simulink model "M_FLCC"  (R2022a)
settings: Solver=ode4  StartTime=0.0  StopTime=100  FixedStep=0.01  RelTol=1e-3
PreLoadFcn:
  | load('BUS_STRUCTURE_FLCC.mat');
InitFcn:
  | load('BUS_STRUCTURE_FLCC.mat');
undefined symbols (not defined in the file or in its folder): f16data
libraries: sharedtransform x6, simulink_extras x4, aerolibatmos2 x1
(part 2 of 2)

== matlab function M_FLCC/FlightController/AttitudeOuterLoop/Auto_Longitudinal/PITCH_AGCAS_PARS/HoldHeight/fcnQuatAttitudeController ==
  data: quat input; qCmd output; quat_sp input; pqr input; beta input; tick input; dt input
function qCmd = fcnQuatAttitudeController(quat, quat_sp, pqr, beta, tick, dt)
%fcnQuatAttitudeController
%
% -- Input --
% quat : quaternion vector (1-by-4 column vector of real numbers)
% quat_sp : (set point) quaternion vector (1-by-4 column vector of real numbers)
% -- Output --
% pqrCmd : angular rate command (3-by-1 column vector of real numbers)

persistent firstRun prev_quat_err prevTick
if isempty(prev_quat_err)
    prev_quat_err = [1, 0, 0, 0];
end
if isempty(firstRun)
    firstRun = true;
end
if isempty(prevTick)
    prevTick = uint32(0);
end

% Initialize Integral control term
if (tick - prevTick ) >= uint32(2)
    prev_quat_err = [1, 0, 0, 0];
end

% Intialize
qCmd = 0.0;
quat_err = zeros(1,4);
eul_ypr = zeros(1,3);

% Controller gain
Kp_p = 2.0;
Kp_q = 0.2;
Kd_q = -0.01;
% Kd_q = -0.0;
Kp_r = 0.0;
Kp_beta = -0.03;
D2R = pi/180;

% Attitude error quaternion
quat_err = quatmultiply( quatconj(quat'), quat_sp' );
quat_err = quatnormalize(quat_err);

% Convert a quat_err to axis-angle representation
ang_err = 2 * acos(quat_err(1));
if ( (IsNear(quat_err(1), 1)) || (IsNear(quat_err(1), -1)) )
    u_x = 0.0;
    u_y = 0.0;
    u_z = 0.0;
else
    u_x = quat_err(2) / sqrt(1 - quat_err(1)^2);
    u_y = quat_err(3) / sqrt(1 - quat_err(1)^2);
    u_z = quat_err(4) / sqrt(1 - quat_err(1)^2);
end

% % Choose a shorter rotation ang_err
if (ang_err > pi)
    ang_err = abs(ang_err - 2*pi);
    u_x = -u_x;
    u_y = -u_y;
    u_z = -u_z;
else
end

% Convert the new attitude error from the axis-angle representation back
% to quaternion form
quat_err(1) = cos(ang_err/2);
quat_err(2) = u_x * sin(ang_err/2);
quat_err(3) = u_y * sin(ang_err/2);
quat_err(4) = u_z * sin(ang_err/2);

eul_ypr = quat2eul(quat', 'ZYX');
% % Ensure we have shorter rotation
if (quat_err(1) < 0)
    quat_err(1) = -quat_err(1);
    quat_err(2) = -quat_err(2);
    quat_err(3) = -quat_err(3);
    quat_err(4) = -quat_err(4);
else
end

% Normalize 
quat_err = quatnormalize(quat_err);

% Euler angles from quaternion
eul_ypr = quat2eul(quat', 'ZYX');
rol = eul_ypr(3);
pit = eul_ypr(2);

% Inversion from attitude kinematics
q = pqr(2);
r = pqr(3);

if abs(pit) > 80*D2R
    pTrim = 0;
    qTrim = 0;
else
    pTrim  =  (- (q * sin(rol) * tan(pit)) - (r * cos(rol) * tan(pit)));
    qTrim  =  (   r * tan(rol));
end
% rTrim  =  (   qTrim / tan(phi));
rTrim  = 0;

% Calculate angular rate command
if (firstRun)
    DTerm = [1, 0, 0, 0];
else
    DTerm = (quat_err - prev_quat_err)/dt;
    DTerm(3) = fcnSaturation(DTerm(3), 0.1);
end
pCmd = pTrim + 2 * Kp_p * quat_err(2);
qCmd = qTrim + 2 * Kp_q * quat_err(3) + Kd_q * DTerm(3);
rCmd = rTrim + 2 * Kp_r * quat_err(4) + Kp_beta * (0 - beta);
% pCmd = K_p * quat_err(2);
% qCmd = K_q * quat_err(3);
% rCmd = rTrim + 2 * K_r * quat_err(4) + Kbeta * (0 - beta);


% Saturate command
plim = 25 * D2R;
qlim = 25 * D2R;
rlim = 20 * D2R;

pCmd = fcnSaturation(pCmd, plim);
qCmd = fcnSaturation(qCmd, qlim);
rCmd = fcnSaturation(rCmd, rlim);

% Output
pqrCmd = [pCmd; qCmd; rCmd];

firstRun = false;
prev_quat_err = quat_err;
prevTick = tick;
end


function in = fcnSaturation(in, lim)

if abs(in)>lim
    in = lim*sign(in);
end

end

== matlab function M_FLCC/FlightController/LeadingEdgeFlapScheduler ==
  data: groundStage input; lefDeg output; alpha input; Ps input; qBar input; lefDegRaw output
function [lefDeg, lefDegRaw]= LeadingEdgeFlapScheduler(groundStage, alpha, Ps, qBar)
%LeadingEdgeFlapScheduler 앞전플랩 명령을 계산한다
% --- INPUT ---
% groundStage: 지상 운동 단계
% ALPHA: 받음각 (deg)
% Ps: 정압 (Pa)
% qBar: 동압 (Pa)
% --- OUTPUT ---
% lefDeg: 앞전플랩 명령 (deg)

% Initialize output
lefDeg = 0.0;
RAD2DEG = 180/pi;

if ( (groundStage >= uint8(2)) && (groundStage <= uint8(5)) )
    % 50%
    lefDeg = 12.5;
else
    if abs(qBar) < 0.1
        lefDeg = 0.0;
    else
        lefDeg = 1.38 * (alpha*RAD2DEG) - 9.05 * (Ps/qBar) + 1.45;
    end
end
lefDegRaw = lefDeg;
lefDeg = fcnSaturation(lefDeg, 0, 25);

end

function out = fcnSaturation(in, lower, upper)

if in > upper
    out = upper;
elseif in < lower
    out = lower;
else
    out = in;
end

end

== matlab function M_FLCC/FlightController/ThrustController/FLCC_CalculateDrag ==
  data: CX input; D output; qBar input; Sref input
function D = CalculateDrag(CX, qBar, Sref)

D = -CX*qBar*Sref;

end

== matlab function M_FLCC/FlightController/ThrustController/FLCC_VelController ==
  data: VtCmd input; Throttle_Cmd output; DYN_STATE input; D input; m input; dt input
function Throttle_Cmd = VelController(VtCmd, DYN_STATE, D, m, dt)
persistent intVtc_Vt prevVtc_Vt
if isempty(intVtc_Vt)
    intVtc_Vt  = 0.0;
    prevVtc_Vt = 0.0;
end

% Constants & Macros
GRAV = 9.8;
DEG2RAD = pi/180;

Vt = DYN_STATE.Vt;
the = DYN_STATE.pitch;
alp = DYN_STATE.alpha;
gam = the - alp;

Vtc_Vt = VtCmd - Vt;
intVtc_Vt  = ( intVtc_Vt + (prevVtc_Vt + Vtc_Vt)*dt/2 );
LimIntVtc_Vt = 50;
intVtc_Vt = fcnSaturation(intVtc_Vt, -LimIntVtc_Vt, LimIntVtc_Vt);
prevVtc_Vt = Vtc_Vt;

% FtTrim = 1/cos(alp)*(D + m*Grav*sin(gam));
% FtTerm1 = wn_Vt^2*m/cos(alp)*intVtc_Vt;
% FtTerm2 = -2*Zeta_Vt*wn_Vt*m/cos(alp)*Vt;

tauVt = 0.28;
intVt = 1.2;

if ( abs(alp) < 85*DEG2RAD )
    Kp  = m/tauVt/cos(alp);
else
    Kp  = m/tauVt/cosd(85);
end
Ki  = intVt;
FtTrimD = 1/cos(alp)*(D); 
FtTrimM = 1/cos(alp)*(m*GRAV*sin(gam));
FtTerm1 = Kp*Vtc_Vt;
FtTerm2 = Ki*intVtc_Vt;

FtCmd   = FtTrimD + FtTrimM + FtTerm1 + FtTerm2;

Ft_lb = fcnSaturation(FtCmd / 4.448, 1000, 29000);
Throttle_Cmd = thrust2thtl(Ft_lb);


end


function out = fcnSaturation(in, lower, upper)

if in > upper
    out = upper;
elseif in < lower
    out = lower;
else
    out = in;
end

end

function thtl = thrust2thtl(thrust_lb)
pow = thrust_lb / 29000;

if (pow <= 0.50)
    thtl = pow / 0.6494;
else
    thtl = (1.1738 + pow) / 2.1738;
end
end

== matlab function M_FLCC/FlightController/AttitudeOuterLoop/Auto_LateralDirectional/fcnQuatAttitudeController ==
  data: quat input; pCmd output; quat_sp input; pqr input; beta input; tick input; dt input; rCmd output
function [pCmd, rCmd] = fcnQuatAttitudeController(quat, quat_sp, pqr, beta, tick, dt)
%fcnQuatAttitudeController
%
% -- Input --
% quat : quaternion vector (1-by-4 column vector of real numbers)
% quat_sp : (set point) quaternion vector (1-by-4 column vector of real numbers)
% -- Output --
% pqrCmd : angular rate command (3-by-1 column vector of real numbers)

persistent firstRun prev_quat_err prevTick
if isempty(prev_quat_err)
    prev_quat_err = [1, 0, 0, 0];
end
if isempty(firstRun)
    firstRun = true;
end
if isempty(prevTick)
    prevTick = uint32(0);
end

% Initialize Integral control term
if (tick - prevTick ) >= uint32(2)
    prev_quat_err = [1, 0, 0, 0];
end

% Intialize
pCmd = 0.0;
rCmd = 0.0;
quat_err = [1, 0, 0, 0];
eul_ypr = zeros(1,3);

% Controller gain
Kp_p = 2.0;
Kp_r = 0.0;
Kp_beta = -0.5;
D2R = pi/180;

% Attitude error quaternion
quat_err = quatmultiply( quatconj(quat'), quat_sp' );
quat_err = quatnormalize(quat_err);

% Convert a quat_err to axis-angle representation
ang_err = 2 * acos(quat_err(1));
if ( (IsNear(quat_err(1), 1)) || (IsNear(quat_err(1), -1)) )
    u_x = 0.0;
    u_y = 0.0;
    u_z = 0.0;
else
    u_x = quat_err(2) / sqrt(1 - quat_err(1)^2);
    u_y = quat_err(3) / sqrt(1 - quat_err(1)^2);
    u_z = quat_err(4) / sqrt(1 - quat_err(1)^2);
end

% % Choose a shorter rotation ang_err
if (ang_err > pi)
    ang_err = abs(ang_err - 2*pi);
    u_x = -u_x;
    u_y = -u_y;
    u_z = -u_z;
else
end

% Convert the new attitude error from the axis-angle representation back
% to quaternion form
quat_err(1) = cos(ang_err/2);
quat_err(2) = u_x * sin(ang_err/2);
quat_err(3) = u_y * sin(ang_err/2);
quat_err(4) = u_z * sin(ang_err/2);

eul_ypr = quat2eul(quat', 'ZYX');
% % Ensure we have shorter rotation
if (quat_err(1) < 0)
    quat_err(1) = -quat_err(1);
    quat_err(2) = -quat_err(2);
    quat_err(3) = -quat_err(3);
    quat_err(4) = -quat_err(4);
else
end

% Normalize 
quat_err = quatnormalize(quat_err);

% Euler angles from quaternion
eul_ypr = quat2eul(quat', 'ZYX');
rol = eul_ypr(3);
pit = eul_ypr(2);

% Inversion from attitude kinematics
p = pqr(1);
q = pqr(2);
r = pqr(3);

if abs(pit) > 80*D2R
    pTrim = 0;
else
    pTrim  =  (- (q * sin(rol) * tan(pit)) - (r * cos(rol) * tan(pit)));
end
rTrim  = 0;

pCmd = pTrim + 2 * Kp_p * quat_err(2);
rCmd = rTrim + 2 * Kp_r * quat_err(4) + Kp_beta * (0 - beta);

% Saturate command
plim = 25 * D2R;
rlim = 20 * D2R;
pCmd = fcnSaturation(pCmd, plim);
rCmd = fcnSaturation(rCmd, rlim);

firstRun = false;
prev_quat_err = quat_err;
prevTick = tick;

end


function in = fcnSaturation(in, lim)

if abs(in)>lim
    in = lim*sign(in);
end

end

== matlab function M_FLCC/FlightController/AttitudeOuterLoop/Manual_Longitudinal/Manual_Long ==
  data: STICK input; qCmd output; DYN_STATE input
function qCmd = Manual_Long(STICK, DYN_STATE)
%Manual_Long
% --- Input ---
% --- Output ---
% qCmd: angular rate command along body y-axis

% Intialize output
qCmd = 0.0;

% Rearrange input
rol = DYN_STATE.roll;
pit = DYN_STATE.pitch;
q = DYN_STATE.omY;
r = DYN_STATE.omZ;
pitchStick = STICK.pitchStick;
expo = 0.5;

if ( -0.05 <= pitchStick ) && ( pitchStick <= 0.05 )
    pitchStick = 0;
else
    pitchStick = (expo*pitchStick^3 + (1-expo)*pitchStick);
end


% Stick
pitchStick = fcnSaturation(pitchStick, 1);

% Controller gain
Kp_q_stick = 0.3;
D2R = pi/180;

if abs(pit) > 80*D2R
    qTrim = 0.0;
else
    qTrim  =  (   r * tan(rol));
end

% Calculate angular rate command
qCmd = qTrim + Kp_q_stick * pitchStick;

% Saturate command
qlim = 25 * D2R;
qCmd = fcnSaturation(qCmd, qlim);

end


function in = fcnSaturation(in, lim)

if abs(in)>lim
    in = lim*sign(in);
end

end

== matlab function M_FLCC/FlightController/AttitudeOuterLoop/Auto_Longitudinal/PITCH_AGCAS_PARS/RecoveryPullUp/GetQCmdATF ==
  data: azCmd input; az input; qCmd output; Vt input; tick input; dt input
function qCmd   = GetQCmdATF(azCmd, az, Vt, tick, dt)
%GetQCmdATF
% == INPUT
% azCmd     : Acceleration Z Command (m/s^2)
% az        : Acceleration Z (m/s^2)
% q         : pitch rate (rad/s)
% U0        : Velocity X (m/s)
% dt        : time interval (sec)
% == OUTPUT
% qCmd      : pitch rate command (rad/s)

persistent zeta wn d2r azInt qInt

if isempty(zeta)
    zeta = 0.70;
end
if isempty(wn)
    wn = 6.3;
end
if isempty(d2r)
    d2r = pi/180;
end
if isempty(azInt)
    azInt = 0.0;
end
if isempty(qInt)
    qInt = 0.0;
end

% Initialize 
qCmd = 0.0;

% Pitch angular velocity command shaping ( azCmd -> qCmd )
Kp_az = - 1 / Vt;
Ki_az = - 1 * 0.05 / Vt;

azInt = azInt + (azCmd - az) * dt;
azInt = fcnSaturation(azInt, 20.0);

qCmd = Kp_az * azCmd + Kp_az * (azCmd - az) + Ki_az * azInt;
end

function out = fcnSaturation(in, lim)

if abs(in) > lim
    out = sign(in)*lim;
else
    out = in;
end

end

== matlab function M_FLCC/FlightController/AttitudeOuterLoop/Auto_Longitudinal/PITCH_AGCAS_PARS/ConfigRecoveryStage ==
  data: prevStage input; curStage output; rollRad input; FPARad input; maxFPARad input
function curStage = ConfigRecoveryStage(prevStage, rollRad, FPARad, maxFPARad)
%ConfigRecoveryStage
% Recovery Stage
% 0: At start / or the end
% 1: Roll Recovering
% 2: Roll Recovered. 5G Pull-Up
% 3: Max Flight Path Angle Reached
% 4: Level Recovering
% 5: Level Recovered

persistent timeSpentMaxFPA dt timeSpentLevelRecovering

if (isempty(dt))
    dt = 0.04;
end
if (isempty(timeSpentMaxFPA))
    timeSpentMaxFPA = 0.0;
end
if (isempty(timeSpentLevelRecovering))
    timeSpentLevelRecovering = 0.0;
end

% Constant
DEG2RAD = pi/180;

curStage = prevStage;

if (prevStage == uint8(0))
    curStage = uint8(1);
    timeSpentMaxFPA = 0.0;
    timeSpentLevelRecovering = 0.0;
else
end

maxFPARad = saturate(maxFPARad, 45*DEG2RAD, 85*DEG2RAD);

if ( (prevStage == uint8(1)) || (curStage == uint8(1)) )
    % Roll 안정화가 되면 2로
    if (rollRad < 0.5*DEG2RAD)
        curStage = uint8(2);
    end

elseif (prevStage == uint8(2))
    % Max Flight Path Angle 도달하면, 3으로
    if ( FPARad > maxFPARad )
        curStage = uint8(3);
    end

elseif (prevStage == uint8(3))
    % 최대 비행경로각 도달 후 10초가 경과하면, 4로
    if (timeSpentMaxFPA > 10.0)
        curStage = uint8(4);
        timeSpentMaxFPA = 0.0;
    else
        timeSpentMaxFPA = timeSpentMaxFPA + dt;
    end

elseif (prevStage == uint8(4))
    
    if (timeSpentLevelRecovering > 5.0)
        curStage = uint8(5);
    end
    timeSpentLevelRecovering = timeSpentLevelRecovering + dt;

elseif (prevStage == uint8(5))

    curStage = uint8(0);

end

end


function outVal = saturate(inVal, minVal, maxVal)

outVal = max(minVal, min(inVal, maxVal));

end

== matlab function M_FLCC/FlightController/AttitudeOuterLoop/Auto_Longitudinal/PITCH_AGCAS_PARS/ConfigStageChange ==
  data: curStage input; prevStage input; isStageChanged output
function isStageChanged  = ConfigStageChange(curStage, prevStage)
%ConfigureStageChange

isStageChanged = false;

if prevStage ~= curStage
    
    isStageChanged = true;
    
else
    
end

end

== matlab function M_FLCC/FlightController/AttitudeOuterLoop/Auto_Longitudinal/PITCH_AGCAS_PARS/UpdateHeightReference ==
  data: oldhRef input; h input; newHRef output; isStageChanged input
function newHRef = UpdateHeightReference(oldhRef, h, isStageChanged)
%UpdateHeightReference

if isStageChanged == true
    
    newHRef = h;
    
else
    
    newHRef = oldhRef;
end

== matlab function M_FLCC/FlightController/AttitudeOuterLoop/Auto_Longitudinal/PITCH_ATF/GetQCmdATF ==
  data: azCmd input; az input; qCmd output; U0 input; tick input; dt input
function qCmd   = GetQCmdATF(azCmd, az, U0, tick, dt)
%GetQCmdATF
% == INPUT
% azCmd     : Acceleration Z Command (m/s^2)
% az        : Acceleration Z (m/s^2)
% q         : pitch rate (rad/s)
% U0        : Velocity X (m/s)
% dt        : time interval (sec)
% == OUTPUT
% qCmd      : pitch rate command (rad/s)

persistent zeta wn d2r azInt qInt prevTick

if isempty(zeta)
    zeta = 0.70;
end
if isempty(wn)
    wn = 6.3;
end
if isempty(d2r)
    d2r = pi/180;
end
if isempty(azInt)
    azInt = 0.0;
end
if isempty(qInt)
    qInt = 0.0;
end
if isempty(prevTick)
    prevTick = uint32(0);
end

% Initialize 
qCmd = 0.0;

if (tick - prevTick >= uint32(2))
    azInt = 0.0;
    qInt = 0.0;
end

% Vt Saturation
U0 = max(75.1089, min(U0, 500));

% Pitch angular velocity command shaping ( azCmd -> qCmd )
Kp_az = - 1.0 / U0;
Ki_az = - 1 * 0.05 / U0;

azInt = azInt + (azCmd - az) * dt;
azInt = fcnSaturation(azInt, 20.0);

qCmd = Kp_az * azCmd + Kp_az * (azCmd - az) + Ki_az * azInt;
% qCmd = Kp_az * azCmd + Kp_az * (azCmd - az) + Ki_az * azInt;
end

function out = fcnSaturation(in, lim)

if abs(in) > lim
    out = sign(in)*lim;
else
    out = in;
end

end

== matlab function M_FLCC/FlightController/AngularRateInnerLoop/fcnPQRController ==
  data: elevatorDEG output; pqrDotCmd input; ALPHA input; BETA input; pqr input; qBar input; Sref input; bref input; cref input; Cln_dar input; Clmn_trim input; inertia input; aileronDEG output; CmMat input; alpIdx input; betIdx input; deIdx1 input; dCm_dsMat input; deIdx3 input; rudderDEG output
function [elevatorDEG, aileronDEG, rudderDEG] = fcnPQRController(pqrDotCmd, ALPHA, BETA, pqr, qBar, Sref, bref, cref,...
    Cln_dar, Clmn_trim, inertia, CmMat, alpIdx, betIdx, deIdx1, dCm_dsMat, deIdx3)
% Dynamic Inversion

%% [1] Moment of inertia Matirx
Ib      = [inertia(1), -inertia(4), -inertia(5);...
          -inertia(4),  inertia(2), -inertia(6);...
          -inertia(5), -inertia(6),  inertia(3)];
%                           % Moment of inertia [kg m^2]

%% [2] Moments (L,M,N) required
% Calculate deflection command 

% Detour for divide by zero (near zero speed, dynamic pressure)
qBar = qBar + 1;
if qBar < 2
    aileronDEG = 0.0;
    rudderDEG = 0.0;
    elevatorDEG = 0.0;
    return
end

Clmn_trim = [Clmn_trim(1);Clmn_trim(2);Clmn_trim(3)];
Qinv = blkdiag( 1/(qBar * Sref * bref), 1/(qBar * Sref * cref), 1/(qBar * Sref * bref) );
M_req     = Ib*pqrDotCmd + cross(pqr, Ib*pqr);
Clmn_defl_cmd = (Qinv*M_req - Clmn_trim);

%% Calculate defelction angle of actuators
% Calculate deflection angle of aileron and rudder ( they are linear )
Cln_dar_Mat = [Cln_dar(1), Cln_dar(2);
               Cln_dar(3), Cln_dar(4)];

dadr = Cln_dar_Mat^-1*[Clmn_defl_cmd(1);Clmn_defl_cmd(3)];
aileronDEG = fcnSaturation(dadr(1), -21.5, 21.5);
rudderDEG  = fcnSaturation(dadr(2), -30, 30);
n = 1000;
% Calculate deflection angle of horizontal stabilizer (not linear, hence
% use numerical method (bisection)

elevatorDEG = bisect(Clmn_defl_cmd(2), CmMat, alpIdx, betIdx, deIdx1, dCm_dsMat, deIdx3, ALPHA, BETA, -25, 25, 0.01, n);
elevatorDEG = fcnSaturation(elevatorDEG, -25, 25);

end

function c = bisect(Cm_defl_cmd, CmMat, alpIdx, betIdx, deIdx1, dCm_dsMat, deIdx3, ALPHA, BETA, deMin, deMax, tol, n)
% Bisection method for solving the nonlinear equation  f(x)=0.
iter=0;
% fx_Upper = feval(f,a);
% fx_Lower = feval(f,b);
% fx_Upper = ( interp3(betIdx, alpIdx, deIdx1, CmMat, ALPHA, BETA, deMin) + interp2(deIdx3, alpIdx, dCm_dsMat, deMin, ALPHA) ) - Cm_defl_cmd;
% fx_Lower = ( interp3(betIdx, alpIdx, deIdx1, CmMat, ALPHA, BETA, deMax) + interp2(deIdx3, alpIdx, dCm_dsMat, deMax, ALPHA) ) - Cm_defl_cmd;
fx_Upper = ( interp3(betIdx, alpIdx, deIdx1, CmMat, BETA, ALPHA, deMin) + interp2(deIdx3, alpIdx, dCm_dsMat, deMin, ALPHA) ) - Cm_defl_cmd;
fx_Lower = ( interp3(betIdx, alpIdx, deIdx1, CmMat, BETA, ALPHA, deMax) + interp2(deIdx3, alpIdx, dCm_dsMat, deMax, ALPHA) ) - Cm_defl_cmd;
c   = (deMin + deMax)*0.5;
err = abs(deMax - deMin)*0.5;
% fprintf("fx_Upper: %f, fx_Lower: %f \r\n", fx_Upper, fx_Lower);
% disp('_____________________________________________________________________')
% disp(' iter    a            b           c           f(c)      |b-a|/2  ')
% disp('_____________________________________________________________________')
% fprintf('\n')
if (fx_Upper*fx_Lower<=0)
%     fprintf("fx_Upper: %f, fx_Lower: %f \r\n", fx_Upper, fx_Lower);

    while (err>tol)&&(iter<=n)
        % w = ( interp3(betIdx, alpIdx, deIdx1, CmMat, alp, bet, c) + interp2(deIdx3, alpIdx, dCm_dsMat, c, alp) ) - Cm_defl_cmd;
        w = ( interp3(betIdx, alpIdx, deIdx1, CmMat, BETA, ALPHA, c) + interp2(deIdx3, alpIdx, dCm_dsMat, c, ALPHA) ) - Cm_defl_cmd;
        % fprintf('%2.0f  %10.4f  %10.4f  %12.6f  %10.6f  %10.6f\n',iter,a,b,c,w,err)
        if (w*fx_Upper<0)
            deMax=c; fx_Lower = w;
        end
        if (w*fx_Upper>0)
            deMin=c; fx_Upper = w;
        end
        iter=iter+1;
        c=(deMin+deMax)*0.5;
        err=abs(deMax-deMin)*0.5;
    end
    if (iter>n)
        c = 0.0;
        %       disp('  Method failed to converge')
    end
else
    c = 0.0;
    %    disp('   The method cannot be applied f(a)f(b)>0')
end
end


function out = fcnSaturation(in, lower, upper)

if in > upper
    out = upper;
elseif in < lower
    out = lower;
else
    out = in;
end

end

== matlab function M_FLCC/FlightController/AngularRateInnerLoop/fcnPQRdotCmd ==
  settings: updateMethod=DISCRETE  sampleTime=0.01
  data: pqrCmd input; pqrDotCmd output; pqr input; pitCtrlMode input; rolCtrlMode input; groundStage input; dt input
function pqrDotCmd = fcnPQRdotCmd(pqrCmd, pqr, pitCtrlMode, rolCtrlMode, groundStage, dt)
%fcnPQRdotCmd
persistent prevPitCtrlMode prevRolCtrlMode prevGroundStage pqrInt
if isempty(prevPitCtrlMode)
    prevPitCtrlMode = uint8(0);
end
if isempty(prevRolCtrlMode)
    prevRolCtrlMode = uint8(0);
end
if isempty(prevGroundStage)
    prevGroundStage = uint8(0);
end
if isempty(pqrInt)
    pqrInt = zeros(3, 1);
end

% Initialize when control mode has been chnaged
if prevPitCtrlMode ~= pitCtrlMode
    pqrInt(2) = 0.0;
end
if prevRolCtrlMode ~= rolCtrlMode
    pqrInt(1) = 0.0;
    pqrInt(3) = 0.0;
end
if prevGroundStage ~= groundStage
    pqrInt = zeros(3, 1);
end

pqrDotCmd = zeros(3,1);

% Constant
d2r = pi/180;

% Second-order controller: gain
wn      = [5.000; 5.000; 5.000];
zeta    = [0.907; 0.700; 0.907];

intLim      = 50 * d2r;
pqrErr      = pqrCmd - pqr;
pqrInt      = pqrInt + pqrErr*dt;
pqrInt(1)   = fcnSaturation(pqrInt(1), intLim);
pqrInt(2)   = fcnSaturation(pqrInt(2), intLim);
pqrInt(3)   = fcnSaturation(pqrInt(3), intLim);
pqrDotCmd   = wn.^2 .* pqrInt - 2 * zeta .* wn .* pqr;

% Update persistent variables
prevPitCtrlMode = pitCtrlMode;
prevRolCtrlMode = rolCtrlMode;
prevGroundStage = groundStage;

end

function out = fcnSaturation(in, lim)

if abs(in) > lim
    out = sign(in)*lim;
else
    out = in;
end

end

== matlab function M_FLCC/FlightController/AttitudeOuterLoop/Auto_Longitudinal/ConfigureMFPA ==
  data: maxFlightPathAngle output; maxFlightPathUint16 input
function maxFlightPathAngle = ConfigureMFPA(maxFlightPathUint16)
%ConfigureMFPA
% -- INPUT --
% paramSelected	        boolean GCAWS 파라미터 선택 여부
% maxFlightPathUint16	uint16	회복기동 모델에 적용하는 최대 비행경로각
%                               [45, 60, 75(d), 90] deg
% -- OUTPUT --
% maxFlightPathAngle    double  (5) Max Flight Path Angle (deg)

% Initialize
maxFlightPathAngle = 0.0;

switch maxFlightPathUint16
    case uint16(0)
        maxFlightPathAngle = 45.0;
    case uint16(1)
        maxFlightPathAngle = 60.0;
    case uint16(2)
        maxFlightPathAngle = 75.0;
    case uint16(3)
        maxFlightPathAngle = 90.0;
    otherwise
        maxFlightPathAngle = 90.0;
end

end

== matlab function M_FLCC/InitNUpdateMapCache/InitializeMAP ==
  data: successDTED output; successDVOF output; latDeg input; lonDeg input
function [successDTED, successDVOF] = InitializeMAP(latDeg, lonDeg)
%InitializeMAP

% Persistent variable
persistent firstRun
if isempty(firstRun)
    firstRun = true;
end

% Initialize output
flagDTED = int32(1);
flagDVOF = int32(1);
successDTED = int32(1);
successDVOF = int32(1);
hDEM = 0.0;

if firstRun
    % Path of DTED data
    pathDTED = 'C:\Users\ASCL\Documents\GitHub\DTNS\MAP\MAP_DB';

    % Length of DETD data path
    strLenDTED = int32(strlength(pathDTED));
    
    hDEM = coder.ceval('MAPGetTerrainHeight', latDeg, lonDeg);
    if IsNear(hDEM, -1.0)
        % Call [ InitialMap ] : 맵 폴더 위치 설정
        flagDTED = coder.ceval('InitialMap', pathDTED, strLenDTED );
        successDTED = flagDTED;
        if (~successDTED)
            firstRun = false;
        end
    else
        successDTED = int32(0);
        firstRun = false;       
    end
else
    successDTED = int32(0);
    successDVOF = int32(0);
end

== matlab function M_FLCC/FlightController/AttitudeOuterLoop/Auto_Longitudinal/ConfigureMPUG ==
  data: maxPullUpG output; pullUpGUint16 input
function maxPullUpG = ConfigureMPUG(pullUpGUint16)
%ConfigureMPUG
% -- INPUT --
% pullUpGUint16	        uint16	피치축 회복기동에 적용하는 G Onset Rate 
% -- OUTPUT
% maxPullUpG            double  (1) Max Pull Up G (g)

% Initialize
maxPullUpG = 0.0;

switch pullUpGUint16
    case uint16(0)
        maxPullUpG = 3.0;
    case uint16(1)
        maxPullUpG = 3.5;
    case uint16(2)
        maxPullUpG = 4.0;
    case uint16(3)
        maxPullUpG = 5.0;
    otherwise
        maxPullUpG = 4.0;
end

== matlab function M_FLCC/h0Manager ==
  data: IN_STATE input; IN_PREV_FLCC_STATE input Bus: BUS_FLCC_AP_STATE; OUT_PREV_FLCC_STATE output Bus: BUS_FLCC_AP_STATE; hDEM input double
function OUT_PREV_FLCC_STATE = h0Manager(IN_STATE, IN_PREV_FLCC_STATE, hDEM)
persistent prevTick firstRun
if isempty(prevTick)
    prevTick = uint32(0);
end
if isempty(firstRun)
    firstRun = true;
end

OUT_PREV_FLCC_STATE = IN_PREV_FLCC_STATE;
if (firstRun)
    if (hDEM >= 0)
        OUT_PREV_FLCC_STATE.h0 = hDEM;
        fprintf("h0: %f \r\n", OUT_PREV_FLCC_STATE.h0);
        firstRun = false;
    end
elseif (IN_PREV_FLCC_STATE.tick - prevTick) >= uint32(100)
    prevTick = IN_PREV_FLCC_STATE.tick;
    OUT_PREV_FLCC_STATE.h0  = coder.ceval('MAPGetTerrainHeight', IN_STATE.latitude, IN_STATE.longitude);
    firstRun = false;
else
end

== matlab function M_FLCC/FlightController/AttitudeOuterLoop/Manual_LateralDirectional/Manual_LatDir ==
  data: STICK input; pCmd output; DYN_STATE input; rCmd output
function [pCmd, rCmd] = Manual_LatDir(STICK, DYN_STATE)
%Manual_LatDir
% --- Input ---
% --- Output ---
% pCmd: angular rate command along body x-axis
% rCmd: angular rate command along body z-axis

% Intialize output
pCmd = 0.0;
rCmd = 0.0;

% Rearrange input
rol = DYN_STATE.roll;
pit = DYN_STATE.pitch;
q = DYN_STATE.omY;
r = DYN_STATE.omZ;
rollStick = STICK.rollStick;
yawStick = STICK.yawStick;
beta = DYN_STATE.beta;

% Stick
expo = 0.5;

if ( -0.05 <= rollStick ) && ( rollStick <= 0.05 )
    rollStick = 0;
else
    rollStick = (expo*rollStick^3 + (1-expo)*rollStick);
end
if ( -0.05 <= yawStick ) && ( yawStick <= 0.05 )
    yawStick = 0;
else
    yawStick = (expo*yawStick^3 + (1-expo)*yawStick);
end

rollStick = fcnSaturation(rollStick, 1);
yawStick = fcnSaturation(yawStick, 1);

% Controller gain
Kp_p_stick = 2.0;
Kp_r_stick = 0.1;
Kp_beta = -0.05;
D2R = pi/180;

if abs(pit) > 80*D2R
    pTrim = 0;
%     qTrim = 0;
else
    pTrim  =  (- (q * sin(rol) * tan(pit)) - (r * cos(rol) * tan(pit)));
%     qTrim  =  (   r * tan(rol));
end
% rTrim  =  (   qTrim / tan(phi));
rTrim  = 0;

% Calculate angular rate command
pCmd = pTrim + Kp_p_stick * rollStick;
rCmd = rTrim + Kp_r_stick * yawStick + Kp_beta * (0 - beta);

% Saturate command
plim = 150 * D2R;
rlim = 20 * D2R;

pCmd = fcnSaturation(pCmd, plim);
rCmd = fcnSaturation(rCmd, rlim);

end


function in = fcnSaturation(in, lim)

if abs(in)>lim
    in = lim*sign(in);
end

end

== matlab function M_FLCC/FlightController/AttitudeOuterLoop/Auto_Longitudinal/If Action Subsystem/MATLAB Function ==
  data: pitCtrlMode input; pitchCmdRad output; FLIGHT_CMD input; DYN_STATE input; pitDesDeg input; tick input; dt input
function pitchCmdRad = shapePitchCmd(pitCtrlMode, FLIGHT_CMD, DYN_STATE, pitDesDeg, tick, dt)
%shapePitchCmd
% --- INPUT ---
% pitCtrlMode : [0=OFF] [1=ATT HOLD] [2=ALT HOLD] [3=ATF] 
%               [4=AGCAS] [5=PARS] uint8
% [FLIGHT_CMD]
% .nextAlt : desired altitude [m]
% [DYN_STATE]
% .Vt : current vehicle's total airspeed [deg]
% .beta : sideslip angle
% .alt
% .alpha
% .eulerAtti
% pitDesDeg : desired ptich angle in ATT HOLD mode
% --- Output ---
% pitchCmdRad : pitch command [rad]

persistent hErrInt prevTick hDotInt
if isempty(hErrInt)
    hErrInt = 0.0; 
end
if isempty(prevTick)
    prevTick = uint32(0);
end
if isempty(hDotInt)
    hDotInt = 0.0;
end

% Initialize
pitchCmdRad = 0.0;

% Constant
D2R = pi/180;

% Rearrange
hCmd = FLIGHT_CMD.nextAlt;
alpha = DYN_STATE.alpha;
Vt = DYN_STATE.Vt;
h = DYN_STATE.altitude;
pitch = DYN_STATE.pitch;
hDot = -DYN_STATE.velD;

switch pitCtrlMode
    case uint8(1)
        %% Attitude Hold
        pitchCmdRad = pitDesDeg * D2R;

    case uint8(2)
        %% Altitude Hold
        
        % PI Control gains for altitude controller
        Kh_p = 0.25;
        Kh_i = 0.01;
        KhDot_p = 4.5;
        KhDot_i = 0.5;

        % Initialize Integral control term when switched
        if (tick - prevTick ) >= uint32(2)
            hErrInt = 0.0;
            hDotInt = 0.0;
        end

        % Control error term & limitation
        hLim    = 100;
        hErrLim = 20;
        hDotlim = 30;
        pitLim  = 20*D2R;
        
        hErr    = fcnSaturation(hCmd - h, hLim);
        hErrInt = fcnSaturation(hErrInt + hErr*dt, hErrLim);

        hDotCmd = fcnSaturation(Kh_p*hErr + Kh_i*hErrInt, hDotlim);
        hDotInt = fcnSaturation(hDotInt + (hDotCmd - hDot)*dt, 10);

        if abs(Vt*cos(pitch)) > 10
            gamCmd = (KhDot_p * (hDotCmd - hDot) + KhDot_i * hDotInt) ...
                / (Vt*cos(pitch));
        else
            gamCmd = (KhDot_p * (hDotCmd - hDot) + KhDot_i * hDotInt);
        end

        % Pitch command
        pitchCmdRad  = fcnSaturation(gamCmd + alpha, pitLim);
        
        % Update Tick
        prevTick = tick;
            
    otherwise
        %% Default
        pitchCmdRad = 0.0;
end

end

%%
function in = fcnSaturation(in, lim)
    if abs(in) > lim
        in = lim*sign(in);
    end
end

== matlab function M_FLCC/FlightController/AttitudeOuterLoop/Auto_LateralDirectional/shapeRollCmd ==
  data: rolCtrlMode input; FLIGHT_CMD input; rollCmdRad output; DYN_STATE input; rolDes input
function rollCmdRad = shapeRollCmd(rolCtrlMode, FLIGHT_CMD, DYN_STATE, rolDes)
%shapeRollCmd
% --- INPUT ---
% rolCtrlMode : [0=OFF(manual), 1=STRG SEL, 2=ATT HOLD, 3=HDG SEL,
%             4=AGCAS, 5=PARS] uint8
% [FLIGHT_CMD]
% .setRoll : desired roll angle in ATT HOLD mode
% .setHeading : desired heading angle in HDG SEL mode
% .nextLat : next latitude [deg]
% .nextLon : next longitude [deg]
% [DYN_STATE]
% .latitude : current vehicle's latitude [deg]
% .longitude : current vehicle's longitude [deg]
% .yaw : current vehicle's heading [deg]
% . Vt : current vehicle's total airspeed [deg]
% --- Output ---
% rollCmdRad : roll command [rad]

% Initialize
rollCmdRad = 0.0;

% Constants
D2R = pi/180;
GRAV = 9.8;
limitRoll = 40 * D2R;

% Rearrange input
setRoll = rolDes;
setHeading = FLIGHT_CMD.setHeading;
nextLat = FLIGHT_CMD.nextLat;
nextLon = FLIGHT_CMD.nextLon;

lat = DYN_STATE.latitude;
lon = DYN_STATE.longitude;
yaw = DYN_STATE.yaw;

Vt = DYN_STATE.Vt;

switch rolCtrlMode
    case uint8(1)
        % [1=STRG SEL] Bank to turn

        % Calculate desired horizontal flight path angle
        % (Assume no sideslip. heading = flight path angle)
        if sqrt((lat-nextLat)^2 + (lon-nextLon)^2) < 0.01
            desiredHdg = yaw;
        else
            nom = cosd(lat)*sind(nextLat) - sind(lat)*cosd(nextLat)*cosd(nextLon - lon);
            den = sind(nextLon - lon) * cosd(nextLat);

            desiredHdg = atan2(den, nom);
        end

        % Initialize heading error
        errorHdg = 0.0;

        % Calculate heading error
        errorTemp = mod(desiredHdg, 360*D2R) - mod(yaw, 360*D2R);

        if (errorTemp <= -180*D2R)
            errorHdg = mod(errorTemp, 360*D2R);
        elseif (errorTemp > 180*D2R)
            errorHdg = -mod(-errorTemp, 360*D2R);
        else
            errorHdg = errorTemp;
        end

        % Calculate heading rate
        hdgDotCmd = 0.25 * errorHdg;
        hdgDotCmd = max(-12*D2R, min(12*D2R, hdgDotCmd));

        % Calculate roll command from heading rate equation
        rollCmdRad = atan( hdgDotCmd * Vt / GRAV );
        rollCmdRad = max(-limitRoll, min(limitRoll, rollCmdRad));

    case uint8(2)
        % [2=ATT HOLD] Hold roll attitude
        rollCmdRad = setRoll * D2R;

    case uint8(3)
        % [3=HDG SEL] Bank to turn
        % Initialize heading error
        errorHdg = 0.0;

        % Calculate heading error
        errorTemp = mod(setHeading*D2R, 360*D2R) - mod(yaw, 360*D2R);

        if (errorTemp <= -180*D2R)
            errorHdg = mod(errorTemp, 360*D2R);
        elseif (errorTemp > 180*D2R)
            errorHdg = -mod(-errorTemp, 360*D2R);
        else
            errorHdg = errorTemp;
        end

        % Calculate heading rate
        hdgDotCmd = 0.25 * errorHdg;
        hdgDotCmd = max(-12*D2R, min(12*D2R, hdgDotCmd));

        % Calculate roll command from heading rate equation
        rollCmdRad = atan( hdgDotCmd * Vt / GRAV );
        rollCmdRad = max(-limitRoll, min(limitRoll, rollCmdRad));


    case {uint8(4), uint8(5)}
        % [4=AGCAS], [5=PARS]
        % Roll Recovery & zero-roll hold for recovery maneuver
        rollCmdRad = 0.0;
        
    otherwise
        % [0=OFF] or Deafualt
        % Stick flight. Autopilot is not working.
        % This is dummy output
        rollCmdRad = 0.0;
end

if isnan(rollCmdRad)
    rollCmdRad = 0.0;
end

end

== matlab function M_FLCC/FlightController/ControlModeManager ==
  data: pitCtrlMode output; FLIGHT_CMD input; PREV_FLCC_STATE input; rolCtrlMode output; pitDesDeg output; rolDesDeg output; inFlying input; groundStage input; collisionWarning input; VtCmd output
function [pitCtrlMode, rolCtrlMode, pitDesDeg, rolDesDeg, VtCmd] = ControlModeManager(FLIGHT_CMD, PREV_FLCC_STATE, inFlying, groundStage, collisionWarning)
%ControlModeManager 현재 항공기 제어 모드를 결정한다
% --- INPUT ---
% FLIGHT_CMD
% PREV_FLCC_STATE: 이전 실행에서의 bus object(BUS_FLCC_AP_STATE)
% inFlying
% groundStage
% collisionWarning
% --- OUTPUT ---
% pitCtrlMode 피치 컨트롤러 작동 모드 (uint8)
%   [0=OFF] [1=ATT HOLD] [2=ALT HOLD] [3=ATF] [4=AGCAS] [5=PARS]
% rolCtrlMode 롤 컨트롤러 작동 모드 (uint8)
%   [0=OFF] [1=STRG SEL] [2=ATT HOLD] [3=HDG SEL] [4=AGCAS] [5=PARS]
% pitDesDeg
% rolDesDeg
% VtCmd
% -------------------------------------------------------------------------

% Initialize output
rolCtrlMode = uint8(0);
pitCtrlMode = uint8(0);
rolDesDeg = 0.0;
pitDesDeg = 0.0;
VtCmd = 0.0;

% Constant
D2R = pi/180;

% Rearrange input
flightMode = FLIGHT_CMD.flightMode;
switchPARS = FLIGHT_CMD.switchPARS;
switchGCAS = FLIGHT_CMD.switchGCAS;
switchTF = FLIGHT_CMD.switchTF;
switchPitch = FLIGHT_CMD.switchPitch;
switchRoll = FLIGHT_CMD.switchRoll;
recoveryStage = PREV_FLCC_STATE.recoveryStage;
rolDesDeg = FLIGHT_CMD.setRoll;
pitDesDeg = FLIGHT_CMD.setPitch;
VtCmd = FLIGHT_CMD.refSpeed;

%% OVERRIDE for Recovery manuever
% FIRST OVERRIDE when Automatic Recovery is already activated
% IF: ON RECOVERY
if (recoveryStage >= uint8(1)) && (recoveryStage < uint8(5))
    % IF: GCAWS
    if switchGCAS == 2
        pitCtrlMode = uint8(4);
        rolCtrlMode = uint8(4);
        % ELSE: PARS (May be...)
    else
        pitCtrlMode = uint8(5);
        rolCtrlMode = uint8(5);
    end
    return
else
end

% SECOND OVERRIDE when AGCAS Recovery Condition is satisfied
% IF: CollisionWarning is activated twice and you are in Auto-GCAWS mode
if ( collisionWarning && ( switchGCAS == 2 ) && (flightMode <= uint8(1)) )
    % Trigger Auto-Recovery
    pitCtrlMode = uint8(4);
    rolCtrlMode = uint8(4);
    return
else
end


%% MANUAL FLIGHT
if ( (flightMode == uint8(0)) || (flightMode == uint8(2)) )
    rolCtrlMode = uint8(0);
    pitCtrlMode = uint8(0);
    return
end

%% AUTO FLIGHT

% ON_GROUND
if (~inFlying)
    rolCtrlMode = uint8(2);
    pitCtrlMode = uint8(1);

    if (groundStage <= uint8(4))
        rolDesDeg = 0.0;
        pitDesDeg = 0.0;
    elseif ( (groundStage > uint8(4)) &&  (groundStage <= uint8(7)) )
        rolDesDeg = 0.0;
        pitDesDeg = 15.0;
    end

    if (groundStage <= uint8(1))
        VtCmd = 0.0;
    elseif (groundStage == uint8(2))
        VtCmd = 10.0;
    elseif (groundStage == uint8(3))
        VtCmd = 100.0;
    elseif (groundStage == uint8(4))
        VtCmd = 100.0;
    elseif (groundStage == uint8(5))
        VtCmd = 150.0;
    elseif (groundStage == uint8(6))
        VtCmd = 150.0;
    elseif (groundStage == uint8(7))
        VtCmd = 150.0;
    end

% IN_FLYING
else
    % Pitch-axis
    if switchPARS == 1
        pitCtrlMode = uint8(5);
    elseif switchTF == 2
        pitCtrlMode = uint8(3);
    elseif (switchTF ~= 2) && (switchPitch == 2)
        pitCtrlMode = uint8(2);

    elseif (switchTF ~= 2) && (switchRoll == 0) && (switchPitch == 1)
        pitCtrlMode = uint8(1);

    elseif (switchPitch == 0)
        pitCtrlMode = uint8(0);
    else
        pitCtrlMode = uint8(0);
    end

    % Roll-axis
    if switchPARS == 1
        rolCtrlMode = uint8(5);
    elseif (switchRoll == 2) && (switchPitch == 2)
        rolCtrlMode = uint8(3);
    elseif (switchRoll == 0) && (switchPitch ~= 0)
        rolCtrlMode = uint8(2);
    elseif (switchRoll == 1) && (switchPitch == 2)
        rolCtrlMode = uint8(1);
    elseif (switchPitch == 0)
        rolCtrlMode = uint8(0);
    else
        rolCtrlMode = uint8(0);
    end
end

end


% CHEATING SHEET ==========================================================
% [ groundStage ]
%               [0 = JUST BOOTED UP]
%               [1 = GROUND IDLE]
%               [2 = TAXING]
%               [3 = READY TAKEOFF]
%               [4 = GROUND ROLL]
%               [5 = ROTATION]
%               [6 = TO AIR TRANSITION]
%               [7 = CLIMBOUT]
%               [8 = IN FLYING]
%               [9 = CRASHES]
% [ FLIGHT_CMD ]
% .switchPARS
%   0	NORM	미입력 상태
%   1	PARS	PARS 절차 수행 트리거
% .switchGCAS
%   0	NOT SELECTED	PGCAS 미선택
%   1	SELECTED        PGCAS 선택 (STBY)
%   2	AUTO GCAS       PGCAS 선택 및 Auto-GCAS 활성화
% .switchTF
%   0	NOT SELECTED	TF 미선택
%   1	SELECTED        TF 선택 (STBY)
%   2	AUTO TF         TF 선택 및 Auto-TF 활성화
% .switchRoll
%   0	ATT HOLD	입력 롤 자세 유지
%   1	STRG SEL	경로점 비행
%   2	HDG SEL     입력 기수방위각 추종
% .switchPitch
%   0	AP OFF      오토파일럿 비활성화
%   1	ATT HOLD	입력 피치자세각 유지 스위치
%   2	ALT HOLD	입력 고도 유지 스위치
%
% [ FLCC_STATE ]
% .recoveryStage
%   0   NORM        회복 기동 수행 아님
%   1   ON RECOVERY 회복 기동 수행중
